simulink model "Memory"  (R2023b)
settings: Solver=VariableStepAuto  StartTime=0.0  StopTime=10.0  RelTol=1e-3
settings Model: Creator=user  LastModifiedBy=user

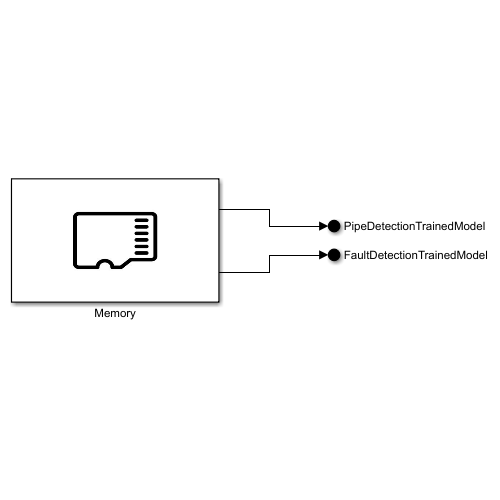
[thumbnail: Simulink's stored preview of the top-level diagram]
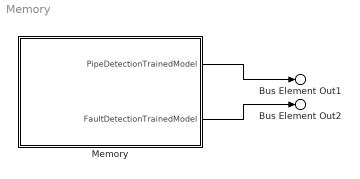
== system Memory ==
  Memory : Subsystem
      mask Display: image('Memory.jpg');
  Bus Element Out1 : Outport  PortName=PipeDetectionTrainedModel
  Bus Element Out2 : Outport  Port=2  PortName=FaultDetectionTrainedModel
  wires:
  Memory/1(PipeDetectionTrainedModel) -> Bus Element Out1/1
  Memory/2(FaultDetectionTrainedModel) -> Bus Element Out2/1

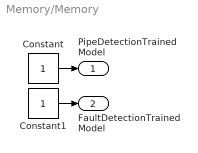
== system Memory/Memory ==
  Constant : Constant
  Constant1 : Constant
  PipeDetectionTrainedModel : Outport
  FaultDetectionTrainedModel : Outport  Port=2
  wires:
  Constant1/1 -> FaultDetectionTrainedModel/1
  Constant/1 -> PipeDetectionTrainedModel/1
